simulink model "Inversor_full_bridge"  (R2015a)
settings: Solver=FixedStepDiscrete  StartTime=0.0  StopTime=0.1  FixedStep=5e-7  MaxStep=5e-7  RelTol=1e-3
libraries: powerlib x11
settings Model: Creator=Leandro  LastModifiedBy=Iury
settings DataIOCC: SignalLoggingSaveFormat=ModelDataLogs
settings DebuggingCC: UnderspecifiedInitializationDetection=Classic  MergeDetectMultiDrivingBlocksExec=none  SolverPrmCheckMsg=warning  FcnCallInpInsideContextMsg=UseLocalSettings  StateNameClashWarn=warning
settings SFSimCC: SimCustomHeaderCode="#include \"controle.h\""  SimUserSources=controle.c
settings GRTTargetCC: CombineOutputUpdateFcns=off  GRTInterface=on

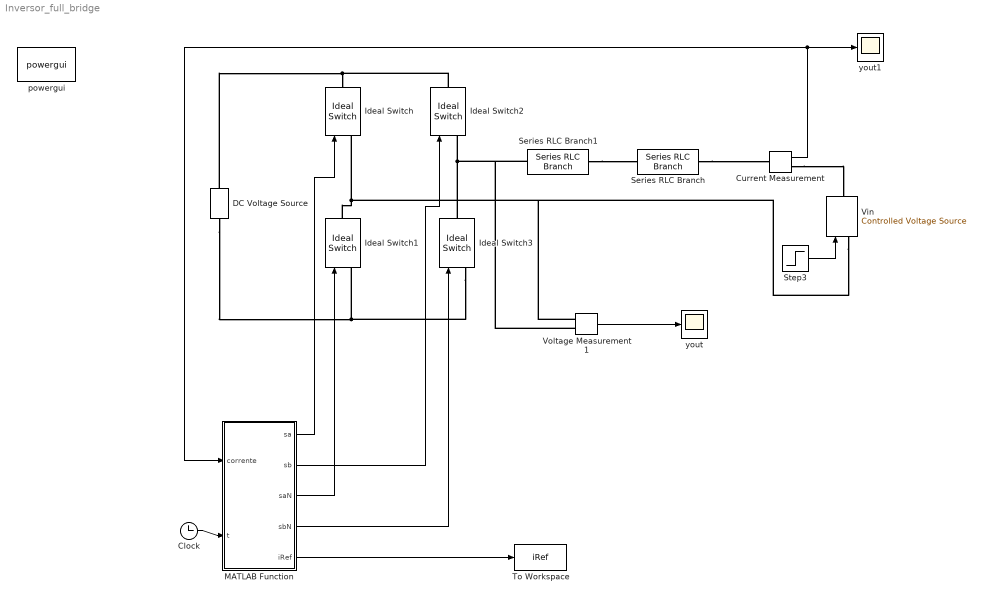
== system Inversor_full_bridge ==
  Clock : Clock
  Current Measurement : powerlib/Measurements/Current Measurement  PhasorSimulation=off  OutputType=Complex  PSBequivalent=0
  DC Voltage Source : powerlib/Electrical Sources/DC Voltage Source  Amplitude=200  Measurements=None
  Ideal Switch{,1..3} (4 alike) : powerlib/Power Electronics/Ideal Switch  Ron=1e-6  Lon=0  IC=0  Rs=1e5  Cs=inf  Measurements=off
  MATLAB Function : MATLAB Function  TreatAsAtomicUnit=on
  Series RLC Branch : powerlib/Elements/Series RLC Branch  LConnTagsString=__new0  RConnTagsString=__new0  BranchType=L  Resistance=0  Inductance=2e-3  SetiL0=off  InitialCurrent=0  Capacitance=1.0  Setx0=off  InitialVoltage=0  Measurements=None
  Series RLC Branch1 : powerlib/Elements/Series RLC Branch  LConnTagsString=__new0  RConnTagsString=__new0  BranchType=R  Resistance=0.1  Inductance=2e-3  SetiL0=off  InitialCurrent=0  Capacitance=1.0  Setx0=off  InitialVoltage=0  Measurements=None
  Step3 : Step  Time=0  After=0  SampleTime=0
  To Workspace : ToWorkspace  VariableName=iRef  SaveFormat=Timeseries  SampleTime=-1
  Vin : powerlib/Electrical Sources/Controlled Voltage Source  Initialize=on  Source_Type=AC  Amplitude=0  Phase=0  Frequency=0  Measurements=None
  Voltage Measurement1 : powerlib/Measurements/Voltage Measurement  PhasorSimulation=off  OutputType=Complex  PSBequivalent=0
  powergui : powerlib/powergui  Priority=1  SimulationMode=Discrete  SolverType=Tustin  SampleTime=5e-7  frequency=60  SPID=on  DisableSnubberDevices=off  DisableRonSwitches=off  DisableVfSwitches=off  SwTol=0  DisplayEquations=off  Interpol=off  methode=off  Ts=0  FunctionMessages=off  echomessages=off  HookPort=off  EnableUseOfTLC=off  x0status=blocks  frequencyindice=0  Pbase=100e6  ErrMax=1e-4  Iterations=50  UnitsV=kV  UnitsW=MW  buscounter=0  RestoreLinks=warning  ResistiveCurrentMeasurement=off  Frange=[0:2:500]  Ylog=off  Xlog=on  ShowGrid=off  save=off  variable=ZData  structure=0  ZoomFFT=off  StartTime=0.0  cycles=1  DisplayStyle=1  fundamental=60  FreqAxis=off  MaxFrequency=1000  frequencyindicesteady=1  RmsSteady=1  display=off
  yout : Scope
      settings: YMin=189.999  YMax=209.999
  yout1 : Scope
      settings: YMin=189.999  YMax=209.999
  wires:
  Current Measurement/1 -> MATLAB Function/1(corrente), yout1/1
  Voltage Measurement1/1 -> yout/1
  Step3/1 -> Vin/1
  Clock/1 -> MATLAB Function/2(t)
  MATLAB Function/5(iRef) -> To Workspace/1
  MATLAB Function/1(sa) -> Ideal Switch/1
  MATLAB Function/2(sb) -> Ideal Switch2/1
  MATLAB Function/3(saN) -> Ideal Switch1/1
  MATLAB Function/4(sbN) -> Ideal Switch3/1
  connections:
  Series RLC Branch/RConn1 -- Current Measurement/LConn1
  Ideal Switch3/RConn1 -- Voltage Measurement1/LConn2 -- Series RLC Branch1/RConn1 -- Ideal Switch2/LConn1
  Ideal Switch2/RConn1 -- DC Voltage Source/RConn1 -- Ideal Switch/RConn1
  Ideal Switch3/LConn1 -- DC Voltage Source/LConn1 -- Ideal Switch1/LConn1
  Ideal Switch1/RConn1 -- Voltage Measurement1/LConn1 -- Vin/LConn1 -- Ideal Switch/LConn1
  Series RLC Branch1/LConn1 -- Series RLC Branch/LConn1
  Current Measurement/RConn1 -- Vin/RConn1

== matlab function Inversor_full_bridge/MATLAB Function ==
  data: sa output; sb output; saN output; sbN output; corrente input; t input; iRef output
function [sa,sb, saN, sbN, iRef]= fcn(corrente, t)

    k1 = -22.626994881450905;
    k2 = -0.561421978901323;
    k3 = 79.163345802203452;
    k4 = -76.791082664183065;

    Sd11 = 0.03125;
    Sd21 = 0;
    Rd11 = 1.998579261776922;
    Rd21 = 1;
    Rd12 = -0.999999980007103;
    Rd22 = 0;

    persistent TPER;

    % Variáveis
    t_ks = 0;	                  		
    n = 0;
    pontos_am = 0;
    modul_ma_k = 0;

    persistent modul_ma_nxt1;
    
    if isempty(modul_ma_nxt1)
        modul_ma_nxt1=0;
    end

    
    v_abf_k = 0;
    ig_k = 0;

    ig_ref_k=0;
    Vcc = 200;
    ig_ref_nxt2 = 0;
    ig_cont_nxt1 = 0;
    ig_ref_amost_ks = 0;
    v_tri = 0;
    sa = 0;
    sb = 0;
    u_ks=0;
    x_ks=0;
    theta_ks=0;
    rho1_ks=0;
    rho2_ks=0;
    Rf = 0.1;
    Lf = 0.005;
    Ig_pk = 10;
    theta = 0;
    w = 376.99;
    
    persistent ig_ref_ks
    
    if isempty(ig_ref_ks)
        ig_ref_ks=0;
    end

    persistent u_k 

    if isempty(u_k)
        u_k=0.5;
    end

    persistent u_nxt1 

    if isempty(u_nxt1)
        u_nxt1=0.5;
    end

    persistent cont

    if isempty(cont)
        cont = 1;
    end

    persistent cont_aux

    if isempty(cont_aux)
        cont_aux = 1;
    end

    persistent rho1_ks_nxt
    if isempty(rho1_ks_nxt)
        rho1_ks_nxt = 0;
    end
    
    persistent rho2_ks_nxt
    if isempty(rho2_ks_nxt)
        rho2_ks_nxt = 0;
    end
    
    Fs = 10000;
    Ts = 1.0e-4;		
    Fsw = 10000;
    Tsw = 1.0e-4;      
    Pontos_fs = 200;  
    Pontos_fsw = 200;

    persistent t_sample;

    if isempty(t_sample)
        t_sample = 200;
    end

    ig_ref_k = Ig_pk*sin(w*t);

    %Controlador
    if t_sample == Pontos_fs 
        ig_k = corrente;

        rho1_ks = rho1_ks_nxt;
        rho2_ks = rho2_ks_nxt;

        ig_ref_ks = ig_ref_k;
        
        x_ks = ig_k;
        t_ks = t_ks + Ts;

        modul_ma_k = modul_ma_nxt1;
        u_k = u_nxt1;

        modul_ma_nxt1 = k1*ig_k + k2*modul_ma_k + k3*rho1_ks + k4*rho2_ks;
        u_nxt1 = (modul_ma_nxt1/(2*Vcc))+0.5;
        
        rho2_ks_nxt = -Sd21*ig_k + 0*modul_ma_k + Rd21*rho1_ks + Rd22*rho2_ks + 0*modul_ma_nxt1 + Sd21 * ig_ref_ks;
        rho1_ks_nxt = -Sd11*ig_k + 0*modul_ma_k + Rd11*rho1_ks + Rd12*rho2_ks + 0*modul_ma_nxt1 + Sd11 * ig_ref_ks;

        t_sample = 0;	
    end

    %Modulador DSP

%     TPER = Pontos_fsw/2;   % PWM simétrico (triangular)
% 
%     if cont_aux < Pontos_fsw
%        cont_aux=cont_aux+1;
%     else
%        cont_aux=1; 
%     end
% 
%     if cont_aux < TPER
%        cont = cont+1;
%     elseif cont_aux >= TPER && cont_aux < Pontos_fsw
%        cont = cont-1;
%     else 
%        cont=1;
%     end
% 
%     if u_k*TPER >= cont
%        sa=1;
%     else
%        sa=0;
%     end

%    sb=1-sa;

    v_tri = 2*asin(sin((2*pi*t/Tsw)-(pi/2)))/pi;
    
    if modul_ma_k/Vcc > v_tri
        sa = 1;
    else
        sa = 0;
    end
        
    if -modul_ma_k/Vcc > v_tri
        sb = 1;
    else
        sb = 0;
    end
    
    saN = 1-sa;
    sbN = 1-sb;
    
    iRef = u_k;

    t_sample = t_sample + 1;
end
